simulink model "ex_water_tank_control"  (R2024b)
settings: Solver=VariableStepAuto  StartTime=0.0  StopTime=1000  RelTol=1e-12
InitFcn:
  | ex_water_tank
values from neighbouring files (symbols this model uses):
  A = [-0.14 0.33 -0.33; 0.1 -0.28 0; 0 1.7 -0.77]    [ex_full_state_feedback.m]    (also in ex_fullfeedback.m; ex_integral_control.m = [-0.14 0.33 -0.33; ex_mi_place.m = [-0.14 0.33 -0.33; ex_mimo_place.m = [-0.14 0.33 -0.33)
  B = [0; 0; -0.025]    [ex_full_state_feedback.m]    (also in ex_fullfeedback.m; ex_integral_control.m; ex_observer.m; ex_pi.m)
  Bv = [1; 0; 0]    [ex_integral_control.m]    (also in ex_mi_place.m = [0; 0; 1]; ex_mimo_place.m = [0; 0; 1]; ex_multi_input_place.m = [0; 0; 1]; ex_pi.m)
  C = [2 0 0]    [ex_full_state_feedback.m]    (also in ex_fullfeedback.m; ex_integral_control.m; ex_mi_place.m; ex_mimo_place.m)
  K = place(A,B,E1(1:3))    [ex_integral_control.m]    (also in ex_specifications.m = place(A,B,E); ex_water.m = K1(:,1:n); ex_water_tank.m = K1(:,1:n))
  Ki = place(Ai,Bi,Ei)    [ex_specifications.m]    (also in ex_water.m = -K1(:,n+1:end); ex_water_tank.m = -K1(:,n+1:end))
  m = 2    [ex_water.m]    (also in ex_water_tank.m)
  n = length(A)    [ex_observer.m]    (also in ex_water.m = 4; ex_water_tank.m = 4)
  u0 = [5; 5]    [ex_water.m]    (also in ex_water_tank.m)
  v = 0.1*sin(8*T)    [ex_integral_control.m]    (also in ex_mi_place.m = 1*ones(size(T)); ex_mimo_place.m = 1*ones(size(T)); ex_pi.m = -1; ex_water.m = 3)
  v0 = [0.0122; 60; 30]    [ex_water.m]    (also in ex_water_tank.m)
  x0 = [1;1;1]    [ex_fullfeedback.m]    (also in ex_water.m = double([sol.x1; sol.x2; sol.x3; sol.x4]); ex_water_tank.m = double([sol.x1; sol.x2; sol.x3; sol.x4]))
settings Model: Creator=Dan  LastModifiedBy=Dan
settings SolverCC: InitialStep=1e-12
settings DataIOCC: SaveFormat=Array
settings OptimizationCC: ReuseModelBlockBuffer=off
settings RTWCC: GPUComputeCapability=3.5

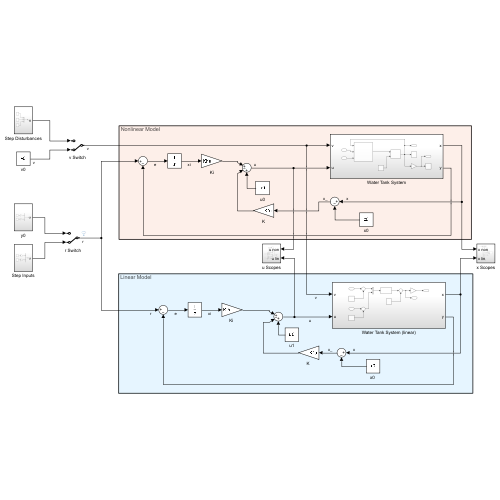
[thumbnail: Simulink's stored preview of the top-level diagram]
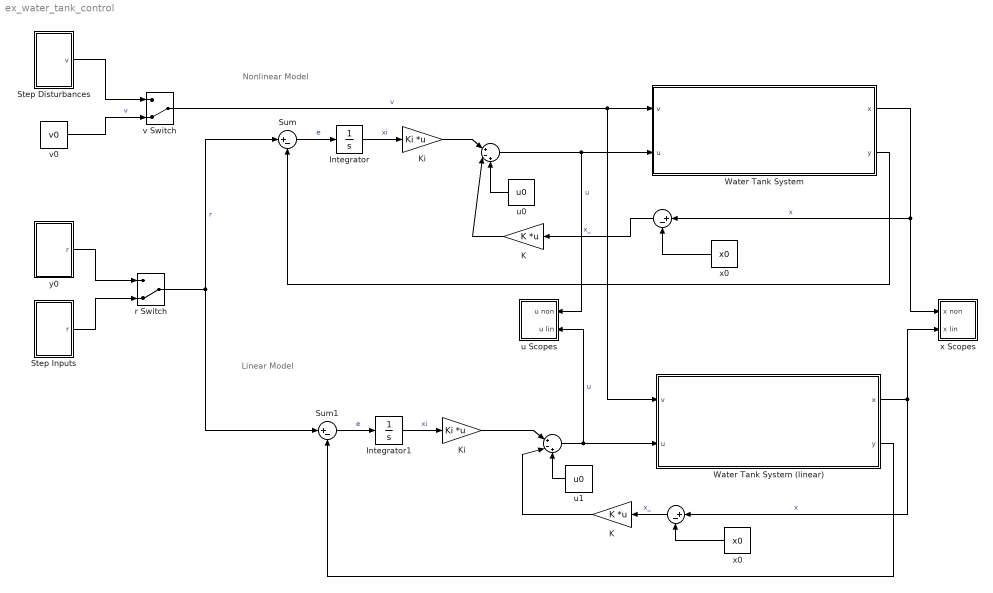
== system ex_water_tank_control ==
  note: Nonlinear Model
  note: Linear Model
  " " : Sum  Inputs=|+-+
  "  " : Sum  Inputs=|+-
  "    " : Sum  Inputs=|+-
  "     " : Sum  Inputs=|+-+
  Integrator : Integrator  InitialCondition=[0;0]
  Integrator1 : Integrator  InitialCondition=[0;0]
  K : Gain  Gain=K  Multiplication=Matrix(K*u)
  "K " : Gain  Gain=K  Multiplication=Matrix(K*u)
  Ki : Gain  Gain=Ki  Multiplication=Matrix(K*u)
  "Ki " : Gain  Gain=Ki  Multiplication=Matrix(K*u)
  Step Disturbances : Subsystem
  Step Inputs : Subsystem
  Sum : Sum  Inputs=|+-
  Sum1 : Sum  Inputs=|+-
  Water Tank System : Subsystem
  Water Tank System (linear) : Subsystem
  r Switch : ManualSwitch  CurrentSetting=0
  u Scopes : Subsystem
  u0 : Constant  Value=u0  VectorParams1D=off
  u1 : Constant  Value=u0  VectorParams1D=off
  v Switch : ManualSwitch  CurrentSetting=0
  v0 : Constant  Value=v0  VectorParams1D=off
  x Scopes : Subsystem
  x0 : Constant  Value=x0  VectorParams1D=off
  "x0 " : Constant  Value=x0  VectorParams1D=off
  y0 : Subsystem
  wires:
  Integrator/1 -> Ki/1  "xi"
  Ki/1 -> " "/1
  " "/1 -> u Scopes/1(u non), Water Tank System/2(u)  "u"
  K/1 -> " "/2
  Water Tank System/1(x) -> "  "/1, x Scopes/1(x non)  "x"
  Sum/1 -> Integrator/1  "e"
  u0/1 -> " "/3
  "  "/1 -> K/1  "x_"
  Water Tank System/2(y) -> Sum/2
  v0/1 -> v Switch/2  "v"
  y0/1(r) -> r Switch/1
  Step Inputs/1(r) -> r Switch/2
  Step Disturbances/1(v) -> v Switch/1
  x0/1 -> "  "/2
  v Switch/1 -> Water Tank System (linear)/1(v), Water Tank System/1(v)  "v"
  "    "/1 -> "K "/1  "x_"
  "K "/1 -> "     "/2
  r Switch/1 -> Sum1/1, Sum/1  "r"
  Integrator1/1 -> "Ki "/1  "xi"
  Sum1/1 -> Integrator1/1  "e"
  Water Tank System (linear)/2(y) -> Sum1/2
  "Ki "/1 -> "     "/1
  u1/1 -> "     "/3
  "     "/1 -> Water Tank System (linear)/2(u), u Scopes/2(u lin)  "u"
  Water Tank System (linear)/1(x) -> "    "/1, x Scopes/2(x lin)  "x"
  "x0 "/1 -> "    "/2

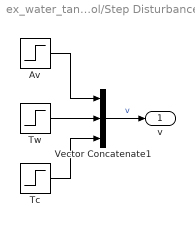
== system ex_water_tank_control/Step Disturbances ==
  Av : Step  Time=100  Before=0.0122  After=0.0134  SampleTime=0
  Tc : Step  Time=700  Before=30  After=10  SampleTime=0
  Tw : Step  Time=400  Before=60  After=95  SampleTime=0
  Vector Concatenate1 : Concatenate  NumInputs=3  Mode=Multidimensional array
  v : Outport
  wires:
  Av/1 -> Vector Concatenate1/1
  Vector Concatenate1/1 -> v/1  "v"
  Tw/1 -> Vector Concatenate1/2
  Tc/1 -> Vector Concatenate1/3

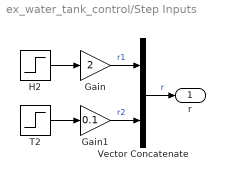
== system ex_water_tank_control/Step Inputs ==
  Gain : Gain  Gain=2
  Gain1 : Gain  Gain=0.1
  H2 : Step  Time=100  Before=x0(2)  After=1.6  SampleTime=0
  T2 : Step  Time=500  Before=x0(4)  After=48  SampleTime=0
  Vector Concatenate : Concatenate  Mode=Multidimensional array
  r : Outport
  wires:
  T2/1 -> Gain1/1
  Gain/1 -> Vector Concatenate/1  "r1"
  H2/1 -> Gain/1
  Vector Concatenate/1 -> r/1  "r"
  Gain1/1 -> Vector Concatenate/2  "r2"

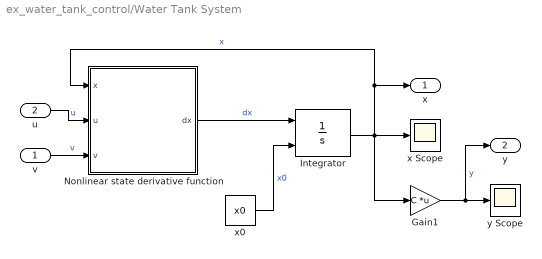
== system ex_water_tank_control/Water Tank System ==
  v : Inport
  u : Inport  Port=2
  Gain1 : Gain  Gain=C  Multiplication=Matrix(K*u)
  Integrator : Integrator  InitialConditionSource=external
  Nonlinear state derivative function : MATLAB Function  TreatAsAtomicUnit=on
  x Scope : Scope
  x0 : Constant  Value=x0  VectorParams1D=off
  y Scope : Scope
  x : Outport
  y : Outport  Port=2
  wires:
  u/1 -> Nonlinear state derivative function/2(u)  "u"
  v/1 -> Nonlinear state derivative function/3(v)  "v"
  Nonlinear state derivative function/1(dx) -> Integrator/1  "dx"
  x0/1 -> Integrator/2  "x0"
  Integrator/1 -> Gain1/1, x/1, Nonlinear state derivative function/1(x), x Scope/1  "x"
  Gain1/1 -> y Scope/1, y/1  "y"

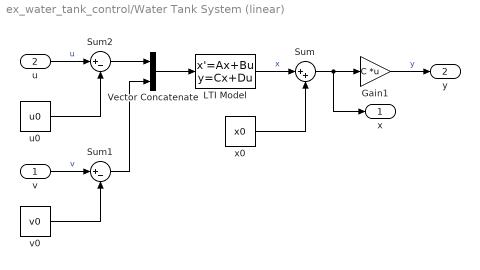
== system ex_water_tank_control/Water Tank System (linear) ==
  v : Inport
  u : Inport  Port=2
  Gain1 : Gain  Gain=C  Multiplication=Matrix(K*u)
  LTI Model : StateSpace  A=A  B=[B,Bv]  C=eye(n)  D=zeros(n,m+v)  InitialCondition=[0; 0; 0; 0]
  Sum : Sum  Inputs=|++
  Sum1 : Sum  Inputs=|+-
  Sum2 : Sum  Inputs=|+-
  Vector Concatenate : Concatenate
  u0 : Constant  Value=u0  VectorParams1D=off
  v0 : Constant  Value=v0  VectorParams1D=off
  x0 : Constant  Value=x0  VectorParams1D=off
  x : Outport
  y : Outport  Port=2
  wires:
  Sum2/1 -> Vector Concatenate/1
  u/1 -> Sum2/1  "u"
  LTI Model/1 -> Sum/1  "x"
  v/1 -> Sum1/1  "v"
  u0/1 -> Sum2/2
  Sum1/1 -> Vector Concatenate/2
  v0/1 -> Sum1/2
  Vector Concatenate/1 -> LTI Model/1
  x0/1 -> Sum/2
  Sum/1 -> x/1, Gain1/1
  Gain1/1 -> y/1  "y"

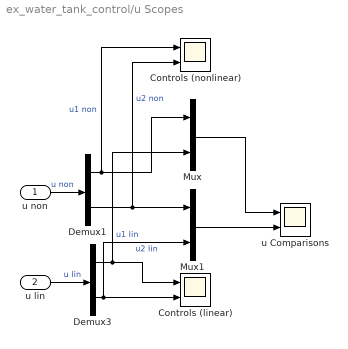
== system ex_water_tank_control/u Scopes ==
  u non : Inport
  u lin : Inport  Port=2
  Controls (linear) : Scope  NumInputPorts=2
  Controls (nonlinear) : Scope  NumInputPorts=2
  Demux1 : Demux  Outputs=2
  Demux3 : Demux  Outputs=2
  Mux : Mux  Inputs=2
  Mux1 : Mux  Inputs=2
  u Comparisons : Scope  NumInputPorts=2
  wires:
  Mux1/1 -> u Comparisons/2
  u non/1 -> Demux1/1  "u non"
  Demux1/1 -> Controls (nonlinear)/1, Mux/1  "u1 non"
  u lin/1 -> Demux3/1  "u lin"
  Demux1/2 -> Controls (nonlinear)/2, Mux1/1  "u2 non"
  Demux3/1 -> Controls (linear)/1, Mux/2  "u1 lin"
  Demux3/2 -> Controls (linear)/2, Mux1/2  "u2 lin"
  Mux/1 -> u Comparisons/1

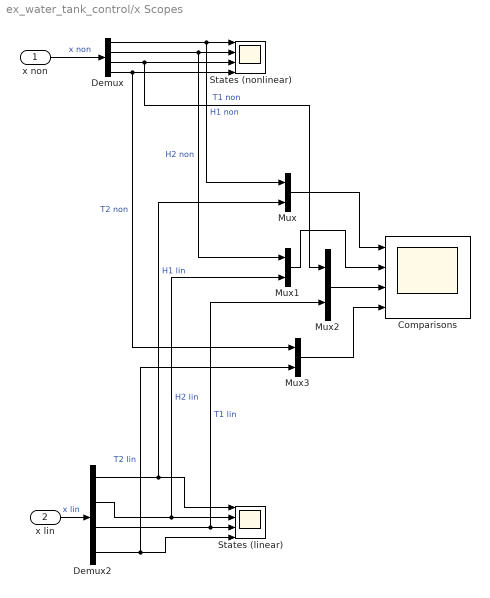
== system ex_water_tank_control/x Scopes ==
  x non : Inport
  x lin : Inport  Port=2
  Comparisons : Scope  NumInputPorts=4
  Demux : Demux
  Demux2 : Demux
  Mux{,1..3} (4 alike) : Mux  Inputs=2
  States (linear) : Scope  NumInputPorts=4
  States (nonlinear) : Scope  NumInputPorts=4
  wires:
  Demux/1 -> States (nonlinear)/1, Mux/1  "H1 non"
  Demux2/3 -> Mux2/2, States (linear)/3  "T1 lin"
  x lin/1 -> Demux2/1  "x lin"
  Demux/2 -> Mux1/1, States (nonlinear)/2  "H2 non"
  Demux2/2 -> Mux1/2, States (linear)/2  "H2 lin"
  Demux2/4 -> Mux3/2, States (linear)/4  "T2 lin"
  Demux/4 -> Mux3/1, States (nonlinear)/4  "T2 non"
  Demux2/1 -> States (linear)/1, Mux/2  "H1 lin"
  x non/1 -> Demux/1  "x non"
  Demux/3 -> Mux2/1, States (nonlinear)/3  "T1 non"
  Mux/1 -> Comparisons/1
  Mux3/1 -> Comparisons/4
  Mux2/1 -> Comparisons/3
  Mux1/1 -> Comparisons/2

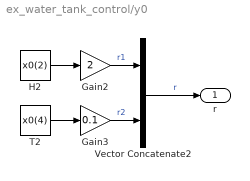
== system ex_water_tank_control/y0 ==
  Gain2 : Gain  Gain=2
  Gain3 : Gain  Gain=0.1
  H2 : Constant  Value=x0(2)
  T2 : Constant  Value=x0(4)
  Vector Concatenate2 : Concatenate  Mode=Multidimensional array
  r : Outport
  wires:
  Vector Concatenate2/1 -> r/1  "r"
  Gain2/1 -> Vector Concatenate2/1  "r1"
  H2/1 -> Gain2/1
  Gain3/1 -> Vector Concatenate2/2  "r2"
  T2/1 -> Gain3/1

== matlab function ex_water_tank_control/Water Tank System/Nonlinear state derivative function ==
  data: x input size=[ 4 1]; u input; dx output; v input
function dx = fcn(x,u,v)

x1 = x(1);
x2 = x(2);
x3 = x(3);
x4 = x(4);

u1 = u(1);
u2 = u(2);

v1 = v(1);
v2 = v(2);
v3 = v(3);

A = 0.785;
ka = 0.004;
C0 = 0.056;
Dv = 2.66;

% state 1 derivative
dx1 = ( ka*(u1 + u2) - C0*sqrt(x1 - x2) )/A;

% state 2 derivative
dx2 = ( C0*sqrt(x1 - x2) - Dv*sqrt(x2)*v1 )/A;

% state 3 derivative
dx3 = ( (v2-x3)*ka*u1 + (v3 - x3)*ka*u2 )/(A*x1);

% state 4 derivative
dx4 = (x3 - x4)*C0*sqrt(x1 - x2)/(A*x2);

% combine
dx = [dx1;dx2;dx3;dx4];
